simulink model "results_comparism"  (R2021a)
settings: Solver=VariableStepAuto  StartTime=0.0  StopTime=100  RelTol=1e-3
undefined symbols (not defined in the file or in its folder): sigbuilder_block
libraries: mpclib x3, simulink x3, cstblocks x1
settings Model: Creator=Owolabi Israel  LastModifiedBy=USER
settings SolverCC: AlgebraicLoopSolver=LineSearch
settings DebuggingCC: SFMachineParentedDataDiag=warning
settings SFSimCC: CustomCodeUndefinedFunction=UseInterfaceOnly

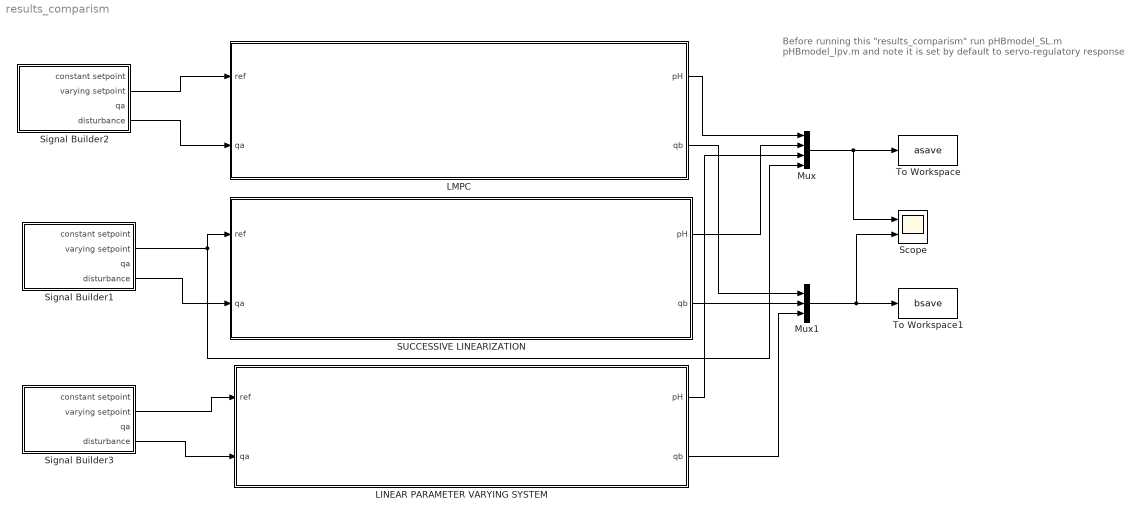
== system results_comparism ==
  note: Before running this "results_comparism"
      | run pHBmodel_SL.m
      | pHBmodel_lpv.m
      | and note it is set by default to servo-regulatory response
  LINEAR PARAMETER VARYING SYSTEM : Subsystem
  LMPC : Subsystem
  Mux : Mux
  Mux1 : Mux  Inputs=3
  SUCCESSIVE LINEARIZATION : Subsystem
  Scope : Scope  NumInputPorts=2
  Signal Builder1 : Subsystem  Tag=STV Subsys  LoadFcn=sigbuilder_block('load');  StartFcn=sigbuilder_block('start');  StopFcn=sigbuilder_block('stop');  ClipboardFcn=sigbuilder_block('clipboard');  mask(Sigbuilder block){tuvar=[0:10]}
      mask help: Simulink:masks:SigbuilderBlock_MD
      mask init:
      | if ~strcmp(get_param(bdroot(gcbh),'SimulationStatus'),'stopped') tuvar = sigbuilder_block('maskInit'); end
      settings: CopyFcn=sigbuilder_block('copy');  DeleteFcn=sigbuilder_block('delete');  ModelCloseFcn=sigbuilder_block('modelClose');  PreSaveFcn=sigbuilder_block('preSave');  PauseFcn=sigbuilder_block('pause');  ContinueFcn=sigbuilder_block('continue');  NameChangeFcn=sigbuilder_block('namechange');  OpenFcn=sigbuilder_block('open',[379.5 6 575 469 ]);  CloseFcn=sigbuilder_block('close');
      mask Display: plot(0, 0, 100, 100,[2, 2, 32, 32, 2], [68, 8, 8, 68, 68],[32, 2], [38, 38], [32, 19, 2],[53, 60, 44], [32, 17, 17, 2],[16, 16, 31, 31]);txt = getActiveGroup(gcbh);text(2, 100, txt,'verticalAlignment', 'top');
  Signal Builder2 : Subsystem  Tag=STV Subsys  LoadFcn=sigbuilder_block('load');  StartFcn=sigbuilder_block('start');  StopFcn=sigbuilder_block('stop');  ClipboardFcn=sigbuilder_block('clipboard');  mask(Sigbuilder block){tuvar=[0:10]}
      mask help: Simulink:masks:SigbuilderBlock_MD
      mask init:
      | if ~strcmp(get_param(bdroot(gcbh),'SimulationStatus'),'stopped') tuvar = sigbuilder_block('maskInit'); end
      settings: CopyFcn=sigbuilder_block('copy');  DeleteFcn=sigbuilder_block('delete');  ModelCloseFcn=sigbuilder_block('modelClose');  PreSaveFcn=sigbuilder_block('preSave');  PauseFcn=sigbuilder_block('pause');  ContinueFcn=sigbuilder_block('continue');  NameChangeFcn=sigbuilder_block('namechange');  OpenFcn=sigbuilder_block('open',[379.5 6 575 469 ]);  CloseFcn=sigbuilder_block('close');
      mask Display: plot(0, 0, 100, 100,[2, 2, 32, 32, 2], [68, 8, 8, 68, 68],[32, 2], [38, 38], [32, 19, 2],[53, 60, 44], [32, 17, 17, 2],[16, 16, 31, 31]);txt = getActiveGroup(gcbh);text(2, 100, txt,'verticalAlignment', 'top');
  Signal Builder3 : Subsystem  Tag=STV Subsys  LoadFcn=sigbuilder_block('load');  StartFcn=sigbuilder_block('start');  StopFcn=sigbuilder_block('stop');  ClipboardFcn=sigbuilder_block('clipboard');  mask(Sigbuilder block){tuvar=[0:10]}
      mask help: Simulink:masks:SigbuilderBlock_MD
      mask init:
      | if ~strcmp(get_param(bdroot(gcbh),'SimulationStatus'),'stopped') tuvar = sigbuilder_block('maskInit'); end
      settings: CopyFcn=sigbuilder_block('copy');  DeleteFcn=sigbuilder_block('delete');  ModelCloseFcn=sigbuilder_block('modelClose');  PreSaveFcn=sigbuilder_block('preSave');  PauseFcn=sigbuilder_block('pause');  ContinueFcn=sigbuilder_block('continue');  NameChangeFcn=sigbuilder_block('namechange');  OpenFcn=sigbuilder_block('open',[379.5 6 575 469 ]);  CloseFcn=sigbuilder_block('close');
      mask Display: plot(0, 0, 100, 100,[2, 2, 32, 32, 2], [68, 8, 8, 68, 68],[32, 2], [38, 38], [32, 19, 2],[53, 60, 44], [32, 17, 17, 2],[16, 16, 31, 31]);txt = getActiveGroup(gcbh);text(2, 100, txt,'verticalAlignment', 'top');
  To Workspace : ToWorkspace  VariableName=asave  SaveFormat=Structure With Time  SampleTime=-1
  To Workspace1 : ToWorkspace  VariableName=bsave  SaveFormat=Structure With Time  SampleTime=-1
  wires:
  Mux/1 -> To Workspace/1, Scope/1
  Mux1/1 -> Scope/2, To Workspace1/1
  LMPC/1(pH) -> Mux/1
  SUCCESSIVE LINEARIZATION/1(pH) -> Mux/2
  LINEAR PARAMETER VARYING SYSTEM/1(pH) -> Mux/3
  LMPC/2(qb) -> Mux1/1
  SUCCESSIVE LINEARIZATION/2(qb) -> Mux1/2
  LINEAR PARAMETER VARYING SYSTEM/2(qb) -> Mux1/3
  Signal Builder2/4(disturbance) -> LMPC/2(qa)
  Signal Builder1/4(disturbance) -> SUCCESSIVE LINEARIZATION/2(qa)
  Signal Builder3/4(disturbance) -> LINEAR PARAMETER VARYING SYSTEM/2(qa)
  Signal Builder2/2(varying setpoint) -> LMPC/1(ref)
  Signal Builder1/2(varying setpoint) -> SUCCESSIVE LINEARIZATION/1(ref), Mux/4
  Signal Builder3/2(varying setpoint) -> LINEAR PARAMETER VARYING SYSTEM/1(ref)

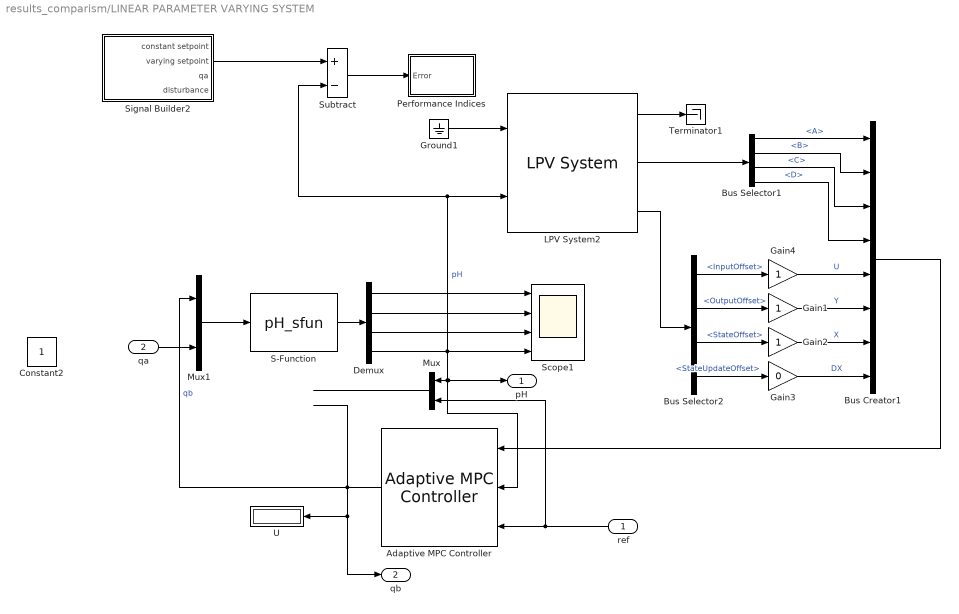
== system results_comparism/LINEAR PARAMETER VARYING SYSTEM ==
  ref : Inport
  qa : Inport  Port=2
  Adaptive MPC Controller : mpclib/Adaptive MPC Controller  SCDEnableBlockLinearizationSpecification=on  mpcobj=mpcobj_lpv  enable_value=0  updateMPCinCallerWorkspace=on  md_inport=off  mv_inport=off  uref_inport=off  return_cost=off  return_mvseq=off  return_qpstatus=off  return_xseq=off  return_state=off  return_ovseq=off  state_inport=off  isltv_plant=off  umin_inport=off  umax_inport=off  ymin_inport=off  ymax_inport=off  cc_inport=off  ywt_inport=off  uwt_inport=off  duwt_inport=off  rhoeps_inport=off  pm_inport=off  MaximumP=10  HorizonChoice=FixedHorizon  BlockDataType=double  SampleTimeInherited=on  switch_inport=off
  Bus Creator1 : BusCreator  Inputs=8
  Bus Selector1 : BusSelector  OutputSignals=A,B,C,D
  Bus Selector2 : BusSelector  OutputSignals=InputOffset,OutputOffset,StateOffset,StateUpdateOffset
  Constant2 : Constant
  Demux : Demux
  Gain1 : Gain
  Gain2 : Gain
  Gain3 : Gain  Gain=0
  Gain4 : Gain
  Ground1 : Ground
  LPV System2 : cstblocks/Linear Parameter Varying/LPV System  sys=lpv  x0=0  uOffset=lpv_u0  yOffset=lpv_y0  xOffset=lpv_x0  opEquilOption=on  dxOffset=0  sysFixedOption=Use the first model in state-space array  sysFixed=[]  AFixed=false  BFixed=false  CFixed=false  DFixed=false  uDelayFixed=true  yDelayFixed=true  iDelayFixed=true  IMethod=Linear  EMethod=Clip  IndexSearch=Binary search  IndexBegin=on  OutputX=off  OutputXdot=off  OutputLTI=on  OutputOP=on  DataType=double  SimMode=Interpreted execution  InitBufferSize=1024  FixedBuffer=off
      settings: SourceProductBaseCode=CT
  Mux : Mux  Inputs=2
  Mux1 : Mux  Inputs=2
  Performance Indices : Subsystem
  S-Function : S-Function  FunctionName=pH_sfun  SFunctionDeploymentMode=off  EnableBusSupport=off
  Scope1 : Scope  NumInputPorts=4
  Signal Builder2 : Subsystem  Tag=STV Subsys  LoadFcn=sigbuilder_block('load');  StartFcn=sigbuilder_block('start');  StopFcn=sigbuilder_block('stop');  ClipboardFcn=sigbuilder_block('clipboard');  mask(Sigbuilder block){tuvar=[0:10]}
      mask help: Simulink:masks:SigbuilderBlock_MD
      mask init:
      | if ~strcmp(get_param(bdroot(gcbh),'SimulationStatus'),'stopped') tuvar = sigbuilder_block('maskInit'); end
      settings: CopyFcn=sigbuilder_block('copy');  DeleteFcn=sigbuilder_block('delete');  ModelCloseFcn=sigbuilder_block('modelClose');  PreSaveFcn=sigbuilder_block('preSave');  PauseFcn=sigbuilder_block('pause');  ContinueFcn=sigbuilder_block('continue');  NameChangeFcn=sigbuilder_block('namechange');  OpenFcn=sigbuilder_block('open',[379.5 6 575 469 ]);  CloseFcn=sigbuilder_block('close');
      mask Display: plot(0, 0, 100, 100,[2, 2, 32, 32, 2], [68, 8, 8, 68, 68],[32, 2], [38, 38], [32, 19, 2],[53, 60, 44], [32, 17, 17, 2],[16, 16, 31, 31]);txt = getActiveGroup(gcbh);text(2, 100, txt,'verticalAlignment', 'top');
  Subtract : Sum  Inputs=+-
  Terminator1 : Terminator
  U : Display
  pH : Outport
  qb : Outport  Port=2
  wires:
  Gain4/1 -> Bus Creator1/5  "U"
  Gain2/1 -> Bus Creator1/7  "X"
  Bus Selector1/1 -> Bus Creator1/1  "<A>"
  Bus Selector1/2 -> Bus Creator1/2  "<B>"
  Subtract/1 -> Performance Indices/1(Error)
  qa/1 -> Mux1/2
  Ground1/1 -> LPV System2/1
  Mux/1 -> ?
  Mux1/1 -> S-Function/1
  Demux/4 -> pH/1, Mux/1, Adaptive MPC Controller/2, Scope1/4, LPV System2/2, Subtract/2  "pH"
  Bus Selector2/4 -> Gain3/1  "<StateUpdateOffset>"
  Bus Creator1/1 -> Adaptive MPC Controller/1
  LPV System2/3 -> Bus Selector2/1
  S-Function/1 -> Demux/1
  LPV System2/1 -> Terminator1/1
  Demux/2 -> Scope1/2
  Adaptive MPC Controller/1 -> Mux1/1, qb/1, U/1  "qb"
  Bus Selector2/1 -> Gain4/1  "<InputOffset>"
  Bus Selector2/3 -> Gain2/1  "<StateOffset>"
  Demux/3 -> Scope1/3
  Bus Selector2/2 -> Gain1/1  "<OutputOffset>"
  Bus Selector1/3 -> Bus Creator1/3  "<C>"
  Demux/1 -> Scope1/1
  Gain1/1 -> Bus Creator1/6  "Y"
  ref/1 -> Mux/2, Adaptive MPC Controller/3
  Gain3/1 -> Bus Creator1/8  "DX"
  Bus Selector1/4 -> Bus Creator1/4  "<D>"
  LPV System2/2 -> Bus Selector1/1
  Signal Builder2/2(varying setpoint) -> Subtract/1

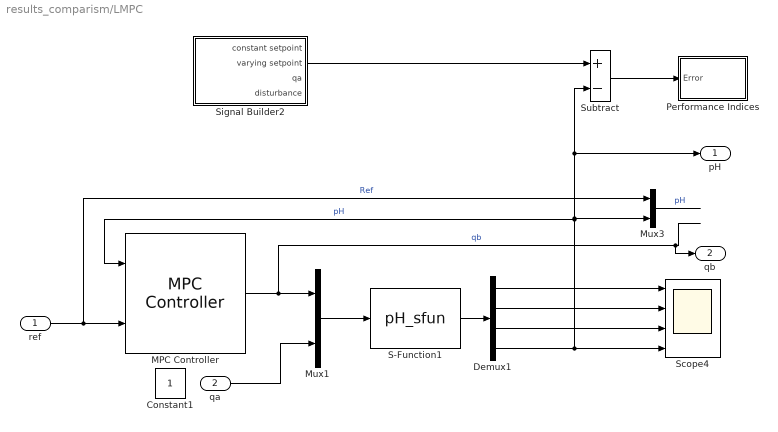
== system results_comparism/LMPC ==
  ref : Inport
  qa : Inport  Port=2
  Constant1 : Constant
  Demux1 : Demux
  MPC Controller : mpclib/MPC Controller  SCDEnableBlockLinearizationSpecification=on  mpcobj=mpcobj_L  is_multiple=0  enable_value=0  return_u0=off  updateMPCinCallerWorkspace=on  md_inport=off  mv_inport=off  uref_inport=off  return_cost=off  return_mvseq=off  return_qpstatus=off  return_xseq=off  return_state=off  return_ovseq=off  state_inport=off  umin_inport=off  umax_inport=off  ymin_inport=off  ymax_inport=off  cc_inport=off  ywt_inport=off  uwt_inport=off  duwt_inport=off  rhoeps_inport=off  pm_inport=off  MaximumP=10  HorizonChoice=FixedHorizon  n_ts=0.1  n_p=100  n_mv=1  n_md=0  n_ud=0  n_mo=1  n_uo=0  BlockDataType=double  SampleTimeInherited=off  switch_inport=off
  Mux1 : Mux  Inputs=2
  Mux3 : Mux  Inputs=2
  Performance Indices : Subsystem
  S-Function1 : S-Function  FunctionName=pH_sfun  SFunctionDeploymentMode=off  EnableBusSupport=off
  Scope4 : Scope  NumInputPorts=4
  Signal Builder2 : Subsystem  Tag=STV Subsys  LoadFcn=sigbuilder_block('load');  StartFcn=sigbuilder_block('start');  StopFcn=sigbuilder_block('stop');  ClipboardFcn=sigbuilder_block('clipboard');  mask(Sigbuilder block){tuvar=[0:10]}
      mask help: Simulink:masks:SigbuilderBlock_MD
      mask init:
      | if ~strcmp(get_param(bdroot(gcbh),'SimulationStatus'),'stopped') tuvar = sigbuilder_block('maskInit'); end
      settings: CopyFcn=sigbuilder_block('copy');  DeleteFcn=sigbuilder_block('delete');  ModelCloseFcn=sigbuilder_block('modelClose');  PreSaveFcn=sigbuilder_block('preSave');  PauseFcn=sigbuilder_block('pause');  ContinueFcn=sigbuilder_block('continue');  NameChangeFcn=sigbuilder_block('namechange');  OpenFcn=sigbuilder_block('open',[379.5 6 575 469 ]);  CloseFcn=sigbuilder_block('close');
      mask Display: plot(0, 0, 100, 100,[2, 2, 32, 32, 2], [68, 8, 8, 68, 68],[32, 2], [38, 38], [32, 19, 2],[53, 60, 44], [32, 17, 17, 2],[16, 16, 31, 31]);txt = getActiveGroup(gcbh);text(2, 100, txt,'verticalAlignment', 'top');
  Subtract : Sum  Inputs=+-
  pH : Outport
  qb : Outport  Port=2
  wires:
  MPC Controller/1 -> Mux1/1, qb/1  "qb"
  Demux1/1 -> Scope4/1
  Demux1/2 -> Scope4/2
  qa/1 -> Mux1/2
  S-Function1/1 -> Demux1/1
  ref/1 -> Mux3/1, MPC Controller/2  "Ref"
  Demux1/3 -> Scope4/3
  Mux3/1 -> ?  "pH"
  Mux1/1 -> S-Function1/1
  Demux1/4 -> Subtract/2, pH/1, Mux3/2, MPC Controller/1, Scope4/4  "pH"
  Subtract/1 -> Performance Indices/1(Error)
  Signal Builder2/2(varying setpoint) -> Subtract/1

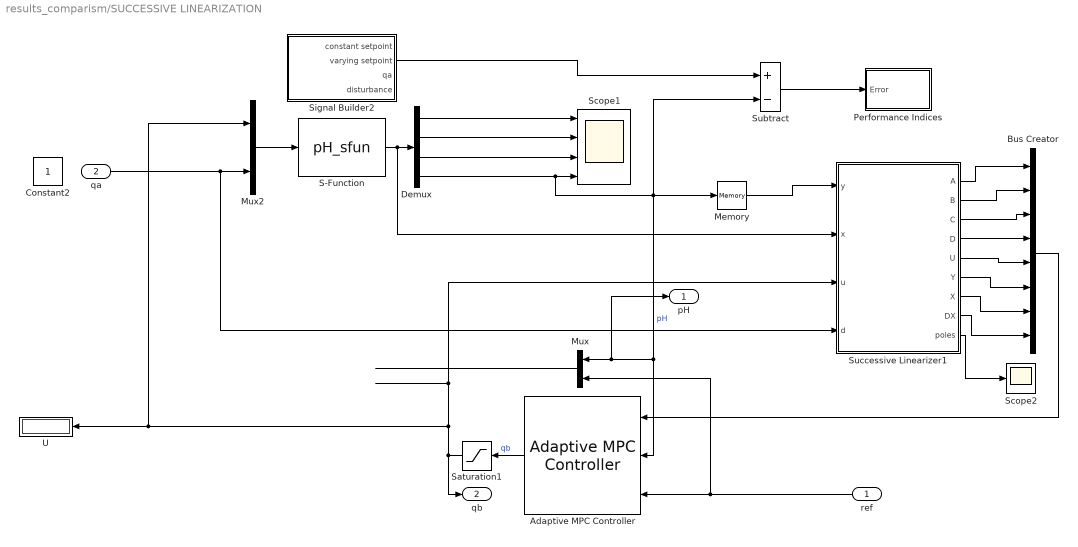
== system results_comparism/SUCCESSIVE LINEARIZATION ==
  ref : Inport
  qa : Inport  Port=2
  Adaptive MPC Controller : mpclib/Adaptive MPC Controller  SCDEnableBlockLinearizationSpecification=on  mpcobj=mpcobj_L  enable_value=0  updateMPCinCallerWorkspace=on  md_inport=off  mv_inport=off  uref_inport=off  return_cost=off  return_mvseq=off  return_qpstatus=off  return_xseq=off  return_state=off  return_ovseq=off  state_inport=off  isltv_plant=off  umin_inport=off  umax_inport=off  ymin_inport=off  ymax_inport=off  cc_inport=off  ywt_inport=off  uwt_inport=off  duwt_inport=off  rhoeps_inport=off  pm_inport=off  MaximumP=10  HorizonChoice=FixedHorizon  BlockDataType=double  SampleTimeInherited=off  switch_inport=off
  Bus Creator : BusCreator  Inputs=8
  Constant2 : Constant
  Demux : Demux
  Memory : Memory  InitialCondition=3
  Mux : Mux  Inputs=2
  Mux2 : Mux  Inputs=2
  Performance Indices : Subsystem
  S-Function : S-Function  FunctionName=pH_sfun  SFunctionDeploymentMode=off  EnableBusSupport=off
  Saturation1 : Saturate  UpperLimit=4  LowerLimit=0
  Scope1 : Scope  NumInputPorts=4
  Scope2 : Scope
  Signal Builder2 : Subsystem  Tag=STV Subsys  LoadFcn=sigbuilder_block('load');  StartFcn=sigbuilder_block('start');  StopFcn=sigbuilder_block('stop');  ClipboardFcn=sigbuilder_block('clipboard');  mask(Sigbuilder block){tuvar=[0:10]}
      mask help: Simulink:masks:SigbuilderBlock_MD
      mask init:
      | if ~strcmp(get_param(bdroot(gcbh),'SimulationStatus'),'stopped') tuvar = sigbuilder_block('maskInit'); end
      settings: CopyFcn=sigbuilder_block('copy');  DeleteFcn=sigbuilder_block('delete');  ModelCloseFcn=sigbuilder_block('modelClose');  PreSaveFcn=sigbuilder_block('preSave');  PauseFcn=sigbuilder_block('pause');  ContinueFcn=sigbuilder_block('continue');  NameChangeFcn=sigbuilder_block('namechange');  OpenFcn=sigbuilder_block('open',[379.5 6 575 469 ]);  CloseFcn=sigbuilder_block('close');
      mask Display: plot(0, 0, 100, 100,[2, 2, 32, 32, 2], [68, 8, 8, 68, 68],[32, 2], [38, 38], [32, 19, 2],[53, 60, 44], [32, 17, 17, 2],[16, 16, 31, 31]);txt = getActiveGroup(gcbh);text(2, 100, txt,'verticalAlignment', 'top');
  Subtract : Sum  Inputs=+-
  Successive Linearizer1 : MATLAB Function  TreatAsAtomicUnit=on  SystemSampleTime=0.5
  U : Display
  pH : Outport
  qb : Outport  Port=2
  wires:
  Successive Linearizer1/9(poles) -> Scope2/1
  S-Function/1 -> Successive Linearizer1/2(x), Demux/1
  Demux/3 -> Scope1/3
  Saturation1/1 -> qb/1, Successive Linearizer1/3(u), U/1, Mux2/1
  Memory/1 -> Successive Linearizer1/1(y)
  Demux/4 -> Adaptive MPC Controller/2, pH/1, Mux/1, Memory/1, Subtract/2, Scope1/4  "pH"
  Adaptive MPC Controller/1 -> Saturation1/1  "qb"
  ref/1 -> Mux/2, Adaptive MPC Controller/3
  Mux2/1 -> S-Function/1
  Demux/2 -> Scope1/2
  Mux/1 -> ?
  Successive Linearizer1/8(DX) -> Bus Creator/8
  Demux/1 -> Scope1/1
  qa/1 -> Successive Linearizer1/4(d), Mux2/2
  Successive Linearizer1/7(X) -> Bus Creator/7
  Bus Creator/1 -> Adaptive MPC Controller/1
  Subtract/1 -> Performance Indices/1(Error)
  Successive Linearizer1/6(Y) -> Bus Creator/6
  Successive Linearizer1/5(U) -> Bus Creator/5
  Successive Linearizer1/4(D) -> Bus Creator/4
  Successive Linearizer1/2(B) -> Bus Creator/2
  Successive Linearizer1/3(C) -> Bus Creator/3
  Successive Linearizer1/1(A) -> Bus Creator/1
  Signal Builder2/2(varying setpoint) -> Subtract/1

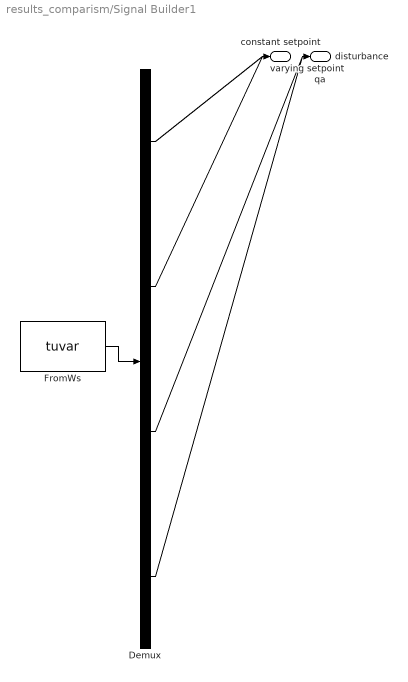
== system results_comparism/Signal Builder1 ==
  Demux : Demux  Tag=STV Demux
      settings: DisplayOption=none
  FromWs : FromWorkspace  Tag=STV FromWs  VariableName=tuvar
      SigBuilderData=|
      | common.afterFinalStr = 'Extrapolate'
      | common.sampleTime = 0
      | dataSet(1).timeRange = [0 100]
      | dataSet(1).name = 'Servo'
      | dataSet(2).timeRange = [0 100]
      | dataSet(2).name = 'Regulatory'
      | sbobj.Groups(1).Name = 'Servo'
      | sbobj.Groups(1).Signals(1).Name = 'constant setpoint'
      | sbobj.Groups(1).Signals(1).XData = [0 100]
      | sbobj.Groups(1).Signals(1).YData = [7 7]
      | sbobj.Groups(1).Signals(2).Name = 'varying setpoint'
      | sbobj.Groups(1).Signals(2).XData = [0 10 10 20 20 30 30 40 40 50 50 60 60 70 70 100]
      | sbobj.Groups(1).Signals(2).YData = [3.14776 3.14776 5 5 6 6 7 7 8 8 9 9 10 10 5 5]
      | sbobj.Groups(1).Signals(3).Name = 'qa'
      | sbobj.Groups(1).Signals(3).XData = [0 100]
      | sbobj.Groups(1).Signals(3).YData = [1 1]
      | sbobj.Groups(1).Signals(4).Name = 'disturbance'
      | sbobj.Groups(1).Signals(4).XData = [0 10 10 20 20 30 30 40 40 50 50 60 60 70 70 80 80 90 90 100]
      | sbobj.Groups(1).Signals(4).YData = [1 1 1.5 1.5 1 1 0.5 0.5 1.5 1.5 1 1 0.5 0.5 1.5 1.5 1 1 0.5 0.5]
      | sbobj.Groups(1).TimeRange = [0 100]
      | sbobj.Groups(2).Name = 'Regulatory'
      | sbobj.Groups(2).Signals(1).Name = 'constant setpoint'
      | sbobj.Groups(2).Signals(1).XData = [0 10 10 20 20 30 30 40 40 50 50 100]
      | sbobj.Groups(2).Signals(1).YData = [1 1 1.5 1.5 1 1 0.5 0.5 1.5 1.5 1 1]
      | sbobj.Groups(2).Signals(2).Name = 'varying setpoint'
      | sbobj.Groups(2).Signals(2).XData = [0 100]
      | sbobj.Groups(2).Signals(2).YData = [7.01 7.01]
      | sbobj.Groups(2).Signals(3).Name = 'qa'
      | sbobj.Groups(2).Signals(3).XData = [0 100]
      | sbobj.Groups(2).Signals(3).YData = [0 0]
      | sbobj.Groups(2).Signals(4).Name = 'disturbance'
      | sbobj.Groups(2).Signals(4).XData = [0 100]
      | sbobj.Groups(2).Signals(4).YData = [0 0]
      | sbobj.Groups(2).TimeRange = [0 100]
  constant setpoint : Outport  Tag=STV Outport  VectorParamsAs1DForOutWhenUnconnected=off
  varying setpoint : Outport  Tag=STV Outport  Port=2  VectorParamsAs1DForOutWhenUnconnected=off
  qa : Outport  Tag=STV Outport  Port=3
  disturbance : Outport  Tag=STV Outport  Port=4
  wires:
  FromWs/1 -> Demux/1
  Demux/1 -> constant setpoint/1
  Demux/2 -> varying setpoint/1
  Demux/3 -> qa/1
  Demux/4 -> disturbance/1

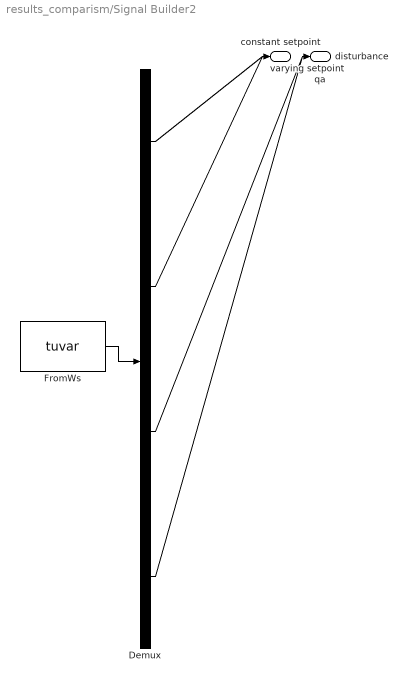
== system results_comparism/Signal Builder2 ==
  Demux : Demux  Tag=STV Demux
      settings: DisplayOption=none
  FromWs : FromWorkspace  Tag=STV FromWs  VariableName=tuvar
      SigBuilderData=|
      | common.afterFinalStr = 'Extrapolate'
      | common.sampleTime = 0
      | dataSet(1).timeRange = [0 100]
      | dataSet(1).name = 'Servo'
      | dataSet(2).timeRange = [0 100]
      | dataSet(2).name = 'Regulatory'
      | sbobj.Groups(1).Name = 'Servo'
      | sbobj.Groups(1).Signals(1).Name = 'constant setpoint'
      | sbobj.Groups(1).Signals(1).XData = [0 100]
      | sbobj.Groups(1).Signals(1).YData = [7 7]
      | sbobj.Groups(1).Signals(2).Name = 'varying setpoint'
      | sbobj.Groups(1).Signals(2).XData = [0 10 10 20 20 30 30 40 40 50 50 60 60 70 70 100]
      | sbobj.Groups(1).Signals(2).YData = [3.14776 3.14776 5 5 6 6 7 7 8 8 9 9 10 10 5 5]
      | sbobj.Groups(1).Signals(3).Name = 'qa'
      | sbobj.Groups(1).Signals(3).XData = [0 100]
      | sbobj.Groups(1).Signals(3).YData = [1 1]
      | sbobj.Groups(1).Signals(4).Name = 'disturbance'
      | sbobj.Groups(1).Signals(4).XData = [0 10 10 20 20 30 30 40 40 50 50 60 60 70 70 80 80 90 90 100]
      | sbobj.Groups(1).Signals(4).YData = [1 1 1.5 1.5 1 1 0.5 0.5 1.5 1.5 1 1 0.5 0.5 1.5 1.5 1 1 0.5 0.5]
      | sbobj.Groups(1).TimeRange = [0 100]
      | sbobj.Groups(2).Name = 'Regulatory'
      | sbobj.Groups(2).Signals(1).Name = 'constant setpoint'
      | sbobj.Groups(2).Signals(1).XData = [0 10 10 20 20 30 30 40 40 50 50 100]
      | sbobj.Groups(2).Signals(1).YData = [1 1 1.5 1.5 1 1 0.5 0.5 1.5 1.5 1 1]
      | sbobj.Groups(2).Signals(2).Name = 'varying setpoint'
      | sbobj.Groups(2).Signals(2).XData = [0 100]
      | sbobj.Groups(2).Signals(2).YData = [7.01 7.01]
      | sbobj.Groups(2).Signals(3).Name = 'qa'
      | sbobj.Groups(2).Signals(3).XData = [0 100]
      | sbobj.Groups(2).Signals(3).YData = [0 0]
      | sbobj.Groups(2).Signals(4).Name = 'disturbance'
      | sbobj.Groups(2).Signals(4).XData = [0 100]
      | sbobj.Groups(2).Signals(4).YData = [0 0]
      | sbobj.Groups(2).TimeRange = [0 100]
  constant setpoint : Outport  Tag=STV Outport  VectorParamsAs1DForOutWhenUnconnected=off
  varying setpoint : Outport  Tag=STV Outport  Port=2  VectorParamsAs1DForOutWhenUnconnected=off
  qa : Outport  Tag=STV Outport  Port=3
  disturbance : Outport  Tag=STV Outport  Port=4
  wires:
  Demux/4 -> disturbance/1
  Demux/3 -> qa/1
  Demux/2 -> varying setpoint/1
  Demux/1 -> constant setpoint/1
  FromWs/1 -> Demux/1

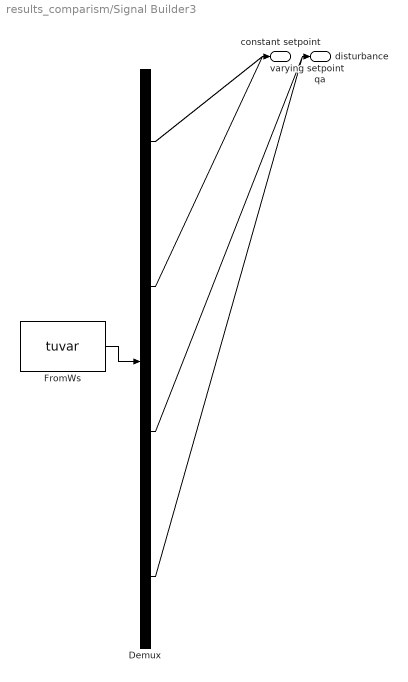
== system results_comparism/Signal Builder3 ==
  Demux : Demux  Tag=STV Demux
      settings: DisplayOption=none
  FromWs : FromWorkspace  Tag=STV FromWs  VariableName=tuvar
      SigBuilderData=|
      | common.afterFinalStr = 'Extrapolate'
      | common.sampleTime = 0
      | dataSet(1).timeRange = [0 100]
      | dataSet(1).name = 'Servo'
      | dataSet(2).timeRange = [0 100]
      | dataSet(2).name = 'Regulatory'
      | sbobj.Groups(1).Name = 'Servo'
      | sbobj.Groups(1).Signals(1).Name = 'constant setpoint'
      | sbobj.Groups(1).Signals(1).XData = [0 100]
      | sbobj.Groups(1).Signals(1).YData = [7 7]
      | sbobj.Groups(1).Signals(2).Name = 'varying setpoint'
      | sbobj.Groups(1).Signals(2).XData = [0 10 10 20 20 30 30 40 40 50 50 60 60 70 70 100]
      | sbobj.Groups(1).Signals(2).YData = [3.14776 3.14776 5 5 6 6 7 7 8 8 9 9 10 10 5 5]
      | sbobj.Groups(1).Signals(3).Name = 'qa'
      | sbobj.Groups(1).Signals(3).XData = [0 100]
      | sbobj.Groups(1).Signals(3).YData = [1 1]
      | sbobj.Groups(1).Signals(4).Name = 'disturbance'
      | sbobj.Groups(1).Signals(4).XData = [0 10 10 20 20 30 30 40 40 50 50 60 60 70 70 80 80 90 90 100]
      | sbobj.Groups(1).Signals(4).YData = [1 1 1.5 1.5 1 1 0.5 0.5 1.5 1.5 1 1 0.5 0.5 1.5 1.5 1 1 0.5 0.5]
      | sbobj.Groups(1).TimeRange = [0 100]
      | sbobj.Groups(2).Name = 'Regulatory'
      | sbobj.Groups(2).Signals(1).Name = 'constant setpoint'
      | sbobj.Groups(2).Signals(1).XData = [0 10 10 20 20 30 30 40 40 50 50 100]
      | sbobj.Groups(2).Signals(1).YData = [1 1 1.5 1.5 1 1 0.5 0.5 1.5 1.5 1 1]
      | sbobj.Groups(2).Signals(2).Name = 'varying setpoint'
      | sbobj.Groups(2).Signals(2).XData = [0 100]
      | sbobj.Groups(2).Signals(2).YData = [7.01 7.01]
      | sbobj.Groups(2).Signals(3).Name = 'qa'
      | sbobj.Groups(2).Signals(3).XData = [0 100]
      | sbobj.Groups(2).Signals(3).YData = [0 0]
      | sbobj.Groups(2).Signals(4).Name = 'disturbance'
      | sbobj.Groups(2).Signals(4).XData = [0 100]
      | sbobj.Groups(2).Signals(4).YData = [0 0]
      | sbobj.Groups(2).TimeRange = [0 100]
  constant setpoint : Outport  Tag=STV Outport  VectorParamsAs1DForOutWhenUnconnected=off
  varying setpoint : Outport  Tag=STV Outport  Port=2  VectorParamsAs1DForOutWhenUnconnected=off
  qa : Outport  Tag=STV Outport  Port=3
  disturbance : Outport  Tag=STV Outport  Port=4
  wires:
  FromWs/1 -> Demux/1
  Demux/1 -> constant setpoint/1
  Demux/2 -> varying setpoint/1
  Demux/3 -> qa/1
  Demux/4 -> disturbance/1

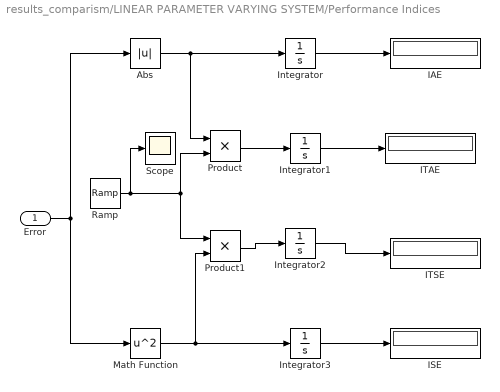
== system results_comparism/LINEAR PARAMETER VARYING SYSTEM/Performance Indices ==
  Error : Inport
  Abs : Abs
  IAE : Display
  ISE : Display
  ITAE : Display
  ITSE : Display
  Integrator{,1..3} (4 alike) : Integrator
  Math Function : Math  Operator=square  SignedPower=on  SaturateOnIntegerOverflow=on
  Product : Product  RndMeth=Zero
  Product1 : Product  RndMeth=Zero
  Ramp : simulink/Sources/Ramp  slope=1  start=0  InitialOutput=0
  Scope : Scope
  wires:
  Error/1 -> Math Function/1, Abs/1
  Abs/1 -> Integrator/1, Product/1
  Integrator/1 -> IAE/1
  Ramp/1 -> Product/2, Product1/1, Scope/1
  Math Function/1 -> Integrator3/1, Product1/2
  Product1/1 -> Integrator2/1
  Product/1 -> Integrator1/1
  Integrator3/1 -> ISE/1
  Integrator2/1 -> ITSE/1
  Integrator1/1 -> ITAE/1

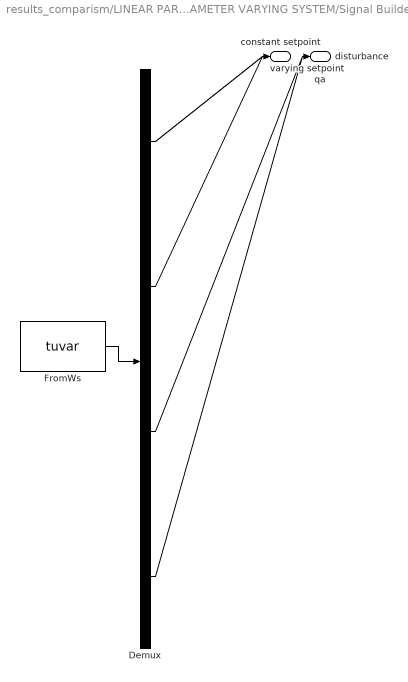
== system results_comparism/LINEAR PARAMETER VARYING SYSTEM/Signal Builder2 ==
  Demux : Demux  Tag=STV Demux
      settings: DisplayOption=none
  FromWs : FromWorkspace  Tag=STV FromWs  VariableName=tuvar
      SigBuilderData=|
      | common.afterFinalStr = 'Extrapolate'
      | common.sampleTime = 0
      | dataSet(1).timeRange = [0 100]
      | dataSet(1).name = 'Servo'
      | dataSet(2).timeRange = [0 100]
      | dataSet(2).name = 'Regulatory'
      | sbobj.Groups(1).Name = 'Servo'
      | sbobj.Groups(1).Signals(1).Name = 'constant setpoint'
      | sbobj.Groups(1).Signals(1).XData = [0 100]
      | sbobj.Groups(1).Signals(1).YData = [7 7]
      | sbobj.Groups(1).Signals(2).Name = 'varying setpoint'
      | sbobj.Groups(1).Signals(2).XData = [0 10 10 20 20 30 30 40 40 50 50 60 60 70 70 100]
      | sbobj.Groups(1).Signals(2).YData = [3.14776 3.14776 5 5 6 6 7 7 8 8 9 9 10 10 5 5]
      | sbobj.Groups(1).Signals(3).Name = 'qa'
      | sbobj.Groups(1).Signals(3).XData = [0 100]
      | sbobj.Groups(1).Signals(3).YData = [1 1]
      | sbobj.Groups(1).Signals(4).Name = 'disturbance'
      | sbobj.Groups(1).Signals(4).XData = [0 10 10 20 20 30 30 40 40 50 50 60 60 70 70 80 80 90 90 100]
      | sbobj.Groups(1).Signals(4).YData = [1 1 1.5 1.5 1 1 0.5 0.5 1.5 1.5 1 1 0.5 0.5 1.5 1.5 1 1 0.5 0.5]
      | sbobj.Groups(1).TimeRange = [0 100]
      | sbobj.Groups(2).Name = 'Regulatory'
      | sbobj.Groups(2).Signals(1).Name = 'constant setpoint'
      | sbobj.Groups(2).Signals(1).XData = [0 10 10 20 20 30 30 40 40 50 50 100]
      | sbobj.Groups(2).Signals(1).YData = [1 1 1.5 1.5 1 1 0.5 0.5 1.5 1.5 1 1]
      | sbobj.Groups(2).Signals(2).Name = 'varying setpoint'
      | sbobj.Groups(2).Signals(2).XData = [0 100]
      | sbobj.Groups(2).Signals(2).YData = [7.01 7.01]
      | sbobj.Groups(2).Signals(3).Name = 'qa'
      | sbobj.Groups(2).Signals(3).XData = [0 100]
      | sbobj.Groups(2).Signals(3).YData = [0 0]
      | sbobj.Groups(2).Signals(4).Name = 'disturbance'
      | sbobj.Groups(2).Signals(4).XData = [0 100]
      | sbobj.Groups(2).Signals(4).YData = [0 0]
      | sbobj.Groups(2).TimeRange = [0 100]
  constant setpoint : Outport  Tag=STV Outport  VectorParamsAs1DForOutWhenUnconnected=off
  varying setpoint : Outport  Tag=STV Outport  Port=2  VectorParamsAs1DForOutWhenUnconnected=off
  qa : Outport  Tag=STV Outport  Port=3
  disturbance : Outport  Tag=STV Outport  Port=4
  wires:
  Demux/4 -> disturbance/1
  Demux/3 -> qa/1
  Demux/2 -> varying setpoint/1
  Demux/1 -> constant setpoint/1
  FromWs/1 -> Demux/1

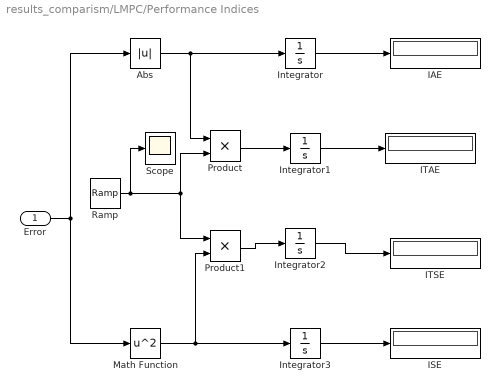
== system results_comparism/LMPC/Performance Indices ==
  Error : Inport
  Abs : Abs
  IAE : Display
  ISE : Display
  ITAE : Display
  ITSE : Display
  Integrator{,1..3} (4 alike) : Integrator
  Math Function : Math  Operator=square  SignedPower=on  SaturateOnIntegerOverflow=on
  Product : Product  RndMeth=Zero
  Product1 : Product  RndMeth=Zero
  Ramp : simulink/Sources/Ramp  slope=1  start=0  InitialOutput=0
  Scope : Scope
  wires:
  Error/1 -> Math Function/1, Abs/1
  Abs/1 -> Integrator/1, Product/1
  Integrator/1 -> IAE/1
  Ramp/1 -> Product/2, Product1/1, Scope/1
  Math Function/1 -> Integrator3/1, Product1/2
  Product1/1 -> Integrator2/1
  Product/1 -> Integrator1/1
  Integrator3/1 -> ISE/1
  Integrator2/1 -> ITSE/1
  Integrator1/1 -> ITAE/1

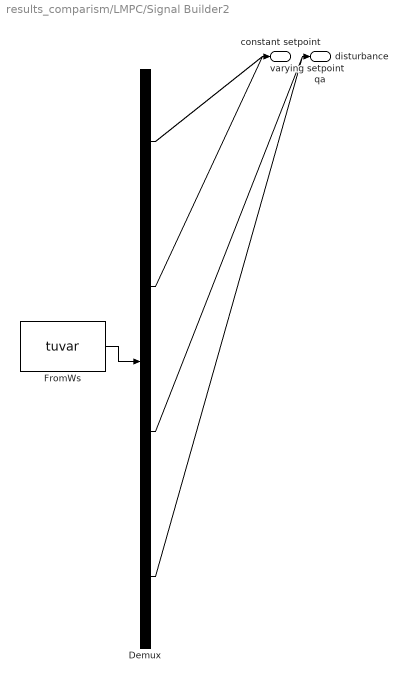
== system results_comparism/LMPC/Signal Builder2 ==
  Demux : Demux  Tag=STV Demux
      settings: DisplayOption=none
  FromWs : FromWorkspace  Tag=STV FromWs  VariableName=tuvar
      SigBuilderData=|
      | common.afterFinalStr = 'Extrapolate'
      | common.sampleTime = 0
      | dataSet(1).timeRange = [0 100]
      | dataSet(1).name = 'Servo'
      | dataSet(2).timeRange = [0 100]
      | dataSet(2).name = 'Regulatory'
      | sbobj.Groups(1).Name = 'Servo'
      | sbobj.Groups(1).Signals(1).Name = 'constant setpoint'
      | sbobj.Groups(1).Signals(1).XData = [0 100]
      | sbobj.Groups(1).Signals(1).YData = [7 7]
      | sbobj.Groups(1).Signals(2).Name = 'varying setpoint'
      | sbobj.Groups(1).Signals(2).XData = [0 10 10 20 20 30 30 40 40 50 50 60 60 70 70 100]
      | sbobj.Groups(1).Signals(2).YData = [3.14776 3.14776 5 5 6 6 7 7 8 8 9 9 10 10 5 5]
      | sbobj.Groups(1).Signals(3).Name = 'qa'
      | sbobj.Groups(1).Signals(3).XData = [0 100]
      | sbobj.Groups(1).Signals(3).YData = [1 1]
      | sbobj.Groups(1).Signals(4).Name = 'disturbance'
      | sbobj.Groups(1).Signals(4).XData = [0 10 10 20 20 30 30 40 40 50 50 60 60 70 70 80 80 90 90 100]
      | sbobj.Groups(1).Signals(4).YData = [1 1 1.5 1.5 1 1 0.5 0.5 1.5 1.5 1 1 0.5 0.5 1.5 1.5 1 1 0.5 0.5]
      | sbobj.Groups(1).TimeRange = [0 100]
      | sbobj.Groups(2).Name = 'Regulatory'
      | sbobj.Groups(2).Signals(1).Name = 'constant setpoint'
      | sbobj.Groups(2).Signals(1).XData = [0 10 10 20 20 30 30 40 40 50 50 100]
      | sbobj.Groups(2).Signals(1).YData = [1 1 1.5 1.5 1 1 0.5 0.5 1.5 1.5 1 1]
      | sbobj.Groups(2).Signals(2).Name = 'varying setpoint'
      | sbobj.Groups(2).Signals(2).XData = [0 100]
      | sbobj.Groups(2).Signals(2).YData = [7.01 7.01]
      | sbobj.Groups(2).Signals(3).Name = 'qa'
      | sbobj.Groups(2).Signals(3).XData = [0 100]
      | sbobj.Groups(2).Signals(3).YData = [0 0]
      | sbobj.Groups(2).Signals(4).Name = 'disturbance'
      | sbobj.Groups(2).Signals(4).XData = [0 100]
      | sbobj.Groups(2).Signals(4).YData = [0 0]
      | sbobj.Groups(2).TimeRange = [0 100]
  constant setpoint : Outport  Tag=STV Outport  VectorParamsAs1DForOutWhenUnconnected=off
  varying setpoint : Outport  Tag=STV Outport  Port=2  VectorParamsAs1DForOutWhenUnconnected=off
  qa : Outport  Tag=STV Outport  Port=3
  disturbance : Outport  Tag=STV Outport  Port=4
  wires:
  Demux/4 -> disturbance/1
  Demux/3 -> qa/1
  Demux/2 -> varying setpoint/1
  Demux/1 -> constant setpoint/1
  FromWs/1 -> Demux/1

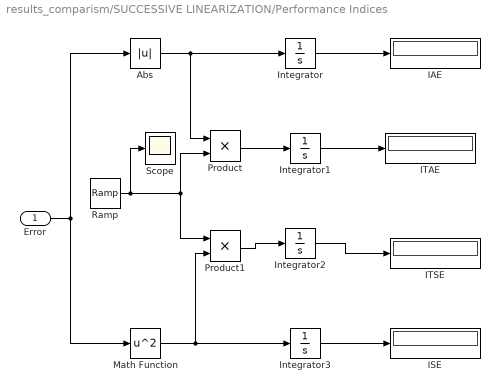
== system results_comparism/SUCCESSIVE LINEARIZATION/Performance Indices ==
  Error : Inport
  Abs : Abs
  IAE : Display
  ISE : Display
  ITAE : Display
  ITSE : Display
  Integrator{,1..3} (4 alike) : Integrator
  Math Function : Math  Operator=square  SignedPower=on  SaturateOnIntegerOverflow=on
  Product : Product  RndMeth=Zero
  Product1 : Product  RndMeth=Zero
  Ramp : simulink/Sources/Ramp  slope=1  start=0  InitialOutput=0
  Scope : Scope
  wires:
  Error/1 -> Math Function/1, Abs/1
  Abs/1 -> Integrator/1, Product/1
  Integrator/1 -> IAE/1
  Ramp/1 -> Product/2, Product1/1, Scope/1
  Math Function/1 -> Integrator3/1, Product1/2
  Product1/1 -> Integrator2/1
  Product/1 -> Integrator1/1
  Integrator3/1 -> ISE/1
  Integrator2/1 -> ITSE/1
  Integrator1/1 -> ITAE/1

== system results_comparism/SUCCESSIVE LINEARIZATION/Signal Builder2 ==
  Demux : Demux  Tag=STV Demux
      settings: DisplayOption=none
  FromWs : FromWorkspace  Tag=STV FromWs  VariableName=tuvar
      SigBuilderData=|
      | common.afterFinalStr = 'Extrapolate'
      | common.sampleTime = 0
      | dataSet(1).timeRange = [0 100]
      | dataSet(1).name = 'Servo'
      | dataSet(2).timeRange = [0 100]
      | dataSet(2).name = 'Regulatory'
      | sbobj.Groups(1).Name = 'Servo'
      | sbobj.Groups(1).Signals(1).Name = 'constant setpoint'
      | sbobj.Groups(1).Signals(1).XData = [0 100]
      | sbobj.Groups(1).Signals(1).YData = [7 7]
      | sbobj.Groups(1).Signals(2).Name = 'varying setpoint'
      | sbobj.Groups(1).Signals(2).XData = [0 10 10 20 20 30 30 40 40 50 50 60 60 70 70 100]
      | sbobj.Groups(1).Signals(2).YData = [3.14776 3.14776 5 5 6 6 7 7 8 8 9 9 10 10 5 5]
      | sbobj.Groups(1).Signals(3).Name = 'qa'
      | sbobj.Groups(1).Signals(3).XData = [0 100]
      | sbobj.Groups(1).Signals(3).YData = [1 1]
      | sbobj.Groups(1).Signals(4).Name = 'disturbance'
      | sbobj.Groups(1).Signals(4).XData = [0 10 10 20 20 30 30 40 40 50 50 60 60 70 70 80 80 90 90 100]
      | sbobj.Groups(1).Signals(4).YData = [1 1 1.5 1.5 1 1 0.5 0.5 1.5 1.5 1 1 0.5 0.5 1.5 1.5 1 1 0.5 0.5]
      | sbobj.Groups(1).TimeRange = [0 100]
      | sbobj.Groups(2).Name = 'Regulatory'
      | sbobj.Groups(2).Signals(1).Name = 'constant setpoint'
      | sbobj.Groups(2).Signals(1).XData = [0 10 10 20 20 30 30 40 40 50 50 100]
      | sbobj.Groups(2).Signals(1).YData = [1 1 1.5 1.5 1 1 0.5 0.5 1.5 1.5 1 1]
      | sbobj.Groups(2).Signals(2).Name = 'varying setpoint'
      | sbobj.Groups(2).Signals(2).XData = [0 100]
      | sbobj.Groups(2).Signals(2).YData = [7.01 7.01]
      | sbobj.Groups(2).Signals(3).Name = 'qa'
      | sbobj.Groups(2).Signals(3).XData = [0 100]
      | sbobj.Groups(2).Signals(3).YData = [0 0]
      | sbobj.Groups(2).Signals(4).Name = 'disturbance'
      | sbobj.Groups(2).Signals(4).XData = [0 100]
      | sbobj.Groups(2).Signals(4).YData = [0 0]
      | sbobj.Groups(2).TimeRange = [0 100]
  constant setpoint : Outport  Tag=STV Outport  VectorParamsAs1DForOutWhenUnconnected=off
  varying setpoint : Outport  Tag=STV Outport  Port=2  VectorParamsAs1DForOutWhenUnconnected=off
  qa : Outport  Tag=STV Outport  Port=3
  disturbance : Outport  Tag=STV Outport  Port=4
  wires:
  Demux/4 -> disturbance/1
  Demux/3 -> qa/1
  Demux/2 -> varying setpoint/1
  Demux/1 -> constant setpoint/1
  FromWs/1 -> Demux/1

== matlab function results_comparism/SUCCESSIVE LINEARIZATION/Successive Linearizer1 ==
  data: y input size=[1,1]; x input; A output size=[3,3]; B output size=[3 1]; C output size=[1,3]; D output size=[1 1]; U output size=[1,1]; Y output size=[1,1]; X output size=[3,1]; DX output size=[3,1]; u input; d input; poles output
function [A, B, C, D, U, Y, X, DX,poles] = fcn(y, x, u, d)

%%%%%%%%%%%%%%%%%%%%%%%%%%%%%%%%%%%%%%%%%%%%%%%%%%%%%%%
%#codegen

% Define constant outputs
Ts = 0.1;
U = u(1) ;
Y = y ;
X = x(1:3) ;



% Analytical linearization of mechanistic CSTR model (continuous time)
% [A, Bo] = getContinuous(T, CA, CAi, Ti, Tc);
[a, b, c, d] = getContinuous(y, x, u, d, Ts)  ;

% Convert continuous to discrete time
% [A, Bo] = getDiscrete(A, Bo, Ts);
[A, Bo, C, D] = getDiscrete(a, b, c, d, Ts)   ;
% Last column of B contains the constant offset contribution.
DX = Bo(:,2);
B = Bo(:,1);
% Compute poles
poles = abs(eig(A));

end

%%%%%%%%%%%%%%%%%%%%%%%%%%%%%%%%%%%%%%%%%%%%%%%%%%%%%
%%%%%%%%%%%%%%%%%%%%%%%%%%%%%%%%%%%

function [a, b, c, d] = getContinuous(y, x, u, d, Ts)




% [A, B, C, D] = get_discrete_model(y, x, u, d, Ts)   ;

%%%%%%%%%%%%%%%%%%%%%%%%%%%%%%%%%%%%%
    qb = u(1);
    qa = d(1);
    
    x1 = x(1);
    x2 = x(2);
    x3 = x(3);
    
    x1i = 0.0012;
    x2i = 0.002;
    x3i = 0.0025;
    kx = 10^-7;
    kw = 10^-14;
    v = 2500e-3;
    
    
    dx1dt = (qa *(x1i - x1) - qb * x1)/v;
    dx2dt = (-qa*x2 + qb*(x2i - x2))/v;
    dx3dt = (-qa*x3 + qb*(x3i - x3))/v;

    %DX = [dx1dt ;  dx2dt ;  dx3dt];

    %%%%%%%%%%%%%%%%%%%%%%%%%%%%%%%%%%
    qb = u(1);
    qa = d(1);
    kx = 10^-7;
    kw = 10^-14;
    
    x1 = x(1);
    x2 = x(2);
    x3 = x(3);
    

    pH = y(1);   
    
    a = [ - (2*qa)/5 - (2*qb)/5,       0,         0;
                    0, - (2*qa)/5 - (2*qb)/5,     0;
                    0,        0, - (2*qa)/5 - (2*qb)/5 ];
          
    b = [ -(2*x1)/5           dx1dt   ; 
        1/1250 - (2*x2)/5     dx2dt  ; 
        1/1000 - (2*x3)/5    dx3dt ]  ;
    
    c = [-1/(log(10)/10^pH + 10^pH*kw*log(10) + (kx*x3*log(10))/(10^pH*kw*(kx/(10^pH*kw) + 1)^2)),...
         1/(log(10)/10^pH + 10^pH*kw*log(10) + (kx*x3*log(10))/(10^pH*kw*(kx/(10^pH*kw) + 1)^2)),...
         -(1/(kx/(10^pH*kw) + 1) - 1)/(log(10)/10^pH + 10^pH*kw*log(10) + (kx*x3*log(10))/(10^pH*kw*(kx/(10^pH*kw) + 1)^2))];
    
    d = 0;
    
    
       
    
    %%%%%%%%%%%%%%%%%%%%%%%%%%%%%%
    
       

end


function [A, B, C, D] = getDiscrete(a, b,c,d, Ts)
% Convert to discrete time
A = expm(a*Ts);
nx = size(b,1);
n = 4;  % Number of points for Simpson's Rule, an even integer >= 2.
% Use Simpson's rule to compute integral(0,Ts){expm(a*s)*ds*b}
h = Ts/n;
Ai = eye(nx) + A;        % First and last terms;
Coef = 2;
for i = 1:n-1
    if Coef == 2
        Coef = 4;
    else
        Coef = 2;
    end
    Ai = Ai + Coef*expm(a*i*h);     % Intermediate terms
end
B = (h/3)*Ai*b;

C = c  ;
D = d ;

end
